simulink model "rpem_16_12_2005"  (Simulink 5.0)
settings: Solver=ode45  StartTime=0.0  StopTime=10.0  RelTol=1e-3
undefined symbols (not defined in the file): ts
libraries: simulink x7, dspmtrx3 x4, dspinverses x1, dsparch4 x1
settings Model: LastModifiedBy=LeO

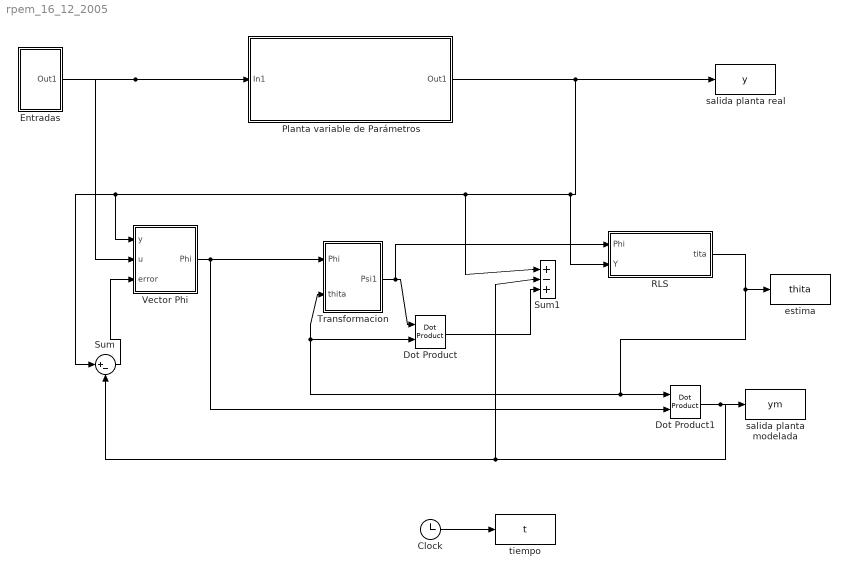
== system rpem_16_12_2005 ==
  Clock : Clock
      settings: Decimation=10
  Dot Product : simulink/Math Operations/Dot Product
  Dot Product1 : simulink/Math Operations/Dot Product
  Entradas : Subsystem
  Planta variable de Parámetros : Subsystem  mask{ruido=0.05, tiempo1=40}
      mask prompts: tiempo1 "tiempo de movimiento de parametros de la planta"
  RLS : Subsystem
  Sum : Sum  Inputs=|+-  SaturateOnIntegerOverflow=on
  Sum1 : Sum  Inputs=|+-+  SaturateOnIntegerOverflow=on
  Transformacion : Subsystem
  Vector Phi : Subsystem  mask{nu=1, ny=3, ne=1, nk=1}
      mask prompts: nu "Nº de u tomadas"; ny "Nº de y tomadas"; ne "Nº de errores tomados"; nk "Nº de retardo"
  estima : ToWorkspace  VariableName=thita  SampleTime=ts  SaveFormat=Array
  "salida planta modelada " : ToWorkspace  VariableName=ym  SampleTime=ts  SaveFormat=Array
  salida planta real : ToWorkspace  VariableName=y  SampleTime=ts  SaveFormat=Array
  "tiempo " : ToWorkspace  VariableName=t  SampleTime=ts  SaveFormat=Array
  wires:
  Entradas/1(Out1) -> Planta variable de Parámetros/1(In1), Vector Phi/2(u)
  Dot Product1/1 -> "salida planta modelada "/1, Sum/2, Sum1/2
  Clock/1 -> "tiempo "/1
  Planta variable de Parámetros/1(Out1) -> salida planta real/1, Vector Phi/1("y "), Sum/1, Sum1/1, RLS/2(Y)
  Transformacion/1(Psi1) -> Dot Product/1, RLS/1("Phi ")
  Vector Phi/1(Phi) -> Dot Product1/2, Transformacion/1(Phi)
  Sum/1 -> Vector Phi/3(error)
  RLS/1(tita) -> estima/1, Transformacion/2(thita), Dot Product/2, Dot Product1/1
  Dot Product/1 -> Sum1/3

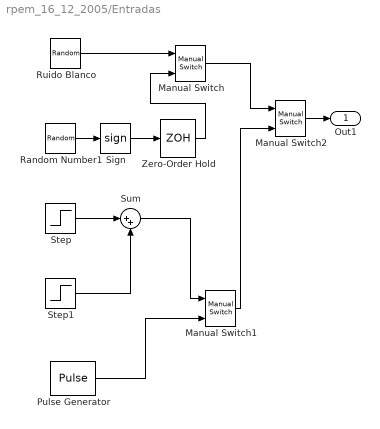
== system rpem_16_12_2005/Entradas ==
  Manual Switch : simulink/Signal Routing/Manual Switch  sw=1  action=0
  Manual Switch1 : simulink/Signal Routing/Manual Switch  sw=1  action=0
  Manual Switch2 : simulink/Signal Routing/Manual Switch  sw=1  action=0
  Pulse Generator : DiscretePulseGenerator  PulseType=Time based  PulseWidth=50
  Random Number1 : RandomNumber  SampleTime=0
  Ruido Blanco : RandomNumber  Variance=20  Seed=12  SampleTime=ts
  Sign : Signum
  Step : Step  Time=10  After=25  SampleTime=0.05
  Step1 : Step  Time=50  After=5  SampleTime=0.05
  Sum : Sum  Inputs=|++  SaturateOnIntegerOverflow=on
  Zero-Order Hold : ZeroOrderHold  SampleTime=0.05
  Out1 : Outport
  wires:
  Sign/1 -> Zero-Order Hold/1
  Random Number1/1 -> Sign/1
  Manual Switch/1 -> Manual Switch2/1
  Ruido Blanco/1 -> Manual Switch/1
  Zero-Order Hold/1 -> Manual Switch/2
  Manual Switch2/1 -> Out1/1
  Step/1 -> Sum/1
  Step1/1 -> Sum/2
  Manual Switch1/1 -> Manual Switch2/2
  Sum/1 -> Manual Switch1/1
  Pulse Generator/1 -> Manual Switch1/2

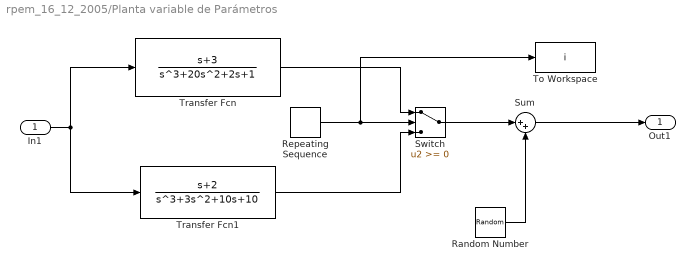
== system rpem_16_12_2005/Planta variable de Parámetros ==
  In1 : Inport
  Random Number : RandomNumber  Variance=ruido  SampleTime=0
  Repeating Sequence : simulink/Sources/Repeating Sequence  rep_seq_t=[0 2*tiempo1]  rep_seq_y=[1 -1 ]
  Sum : Sum  Inputs=|++  SaturateOnIntegerOverflow=on
  Switch : Switch  SaturateOnIntegerOverflow=on
  To Workspace : ToWorkspace  VariableName=i  SampleTime=-1  SaveFormat=Array
  Transfer Fcn : TransferFcn  Numerator=[1 3 ]  Denominator=[1 20 2 1]
  Transfer Fcn1 : TransferFcn  Numerator=[1 2]  Denominator=[1 3 10 10]
  Out1 : Outport
  wires:
  Transfer Fcn/1 -> Switch/1
  Repeating Sequence/1 -> Switch/2, To Workspace/1
  Transfer Fcn1/1 -> Switch/3
  In1/1 -> Transfer Fcn/1, Transfer Fcn1/1
  Switch/1 -> Sum/1
  Sum/1 -> Out1/1
  Random Number/1 -> Sum/2

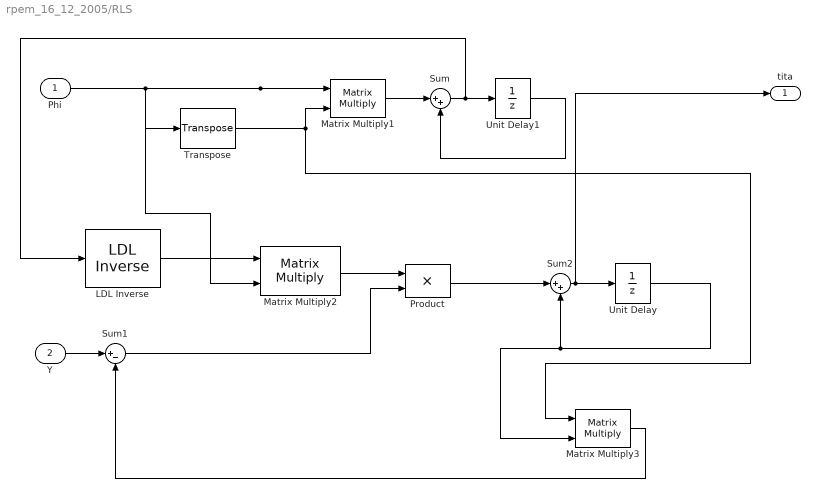
== system rpem_16_12_2005/RLS ==
  "Phi " : Inport  SampleTime=ts
  Y : Inport  Port=2  SampleTime=ts
  LDL Inverse : dspinverses/LDL Inverse  errmode=Ignore
  Matrix Multiply1 : dspmtrx3/Matrix Multiply  numInputPorts=2  OptimizationLevel=None
  Matrix Multiply2 : dspmtrx3/Matrix Multiply  numInputPorts=2  OptimizationLevel=None
  Matrix Multiply3 : dspmtrx3/Matrix Multiply  numInputPorts=2  OptimizationLevel=None
  Product : Product  SaturateOnIntegerOverflow=on
  Sum : Sum  Inputs=|++  SaturateOnIntegerOverflow=on
  Sum1 : Sum  Inputs=|+-  SaturateOnIntegerOverflow=on
  Sum2 : Sum  Inputs=|++  SaturateOnIntegerOverflow=on
  Transpose : dspmtrx3/Transpose  Hermitian=off
  Unit Delay : UnitDelay  X0=1*10^-3  SampleTime=ts
  Unit Delay1 : UnitDelay  X0=10^-3  SampleTime=ts
  tita : Outport
  wires:
  "Phi "/1 -> Transpose/1, Matrix Multiply2/2, Matrix Multiply1/1
  Transpose/1 -> Matrix Multiply3/1, Matrix Multiply1/2
  Matrix Multiply1/1 -> Sum/1
  Sum/1 -> Unit Delay1/1, LDL Inverse/1
  Unit Delay1/1 -> Sum/2
  LDL Inverse/1 -> Matrix Multiply2/1
  Sum2/1 -> Unit Delay/1, tita/1
  Y/1 -> Sum1/1
  Matrix Multiply2/1 -> Product/1
  Product/1 -> Sum2/1
  Matrix Multiply3/1 -> Sum1/2
  Sum1/1 -> Product/2
  Unit Delay/1 -> Matrix Multiply3/2, Sum2/2

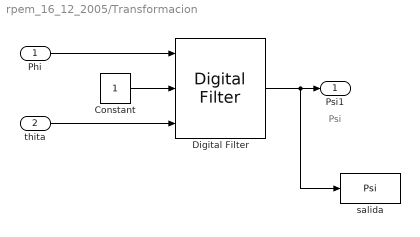
== system rpem_16_12_2005/Transformacion ==
  note: Psi
  Phi : Inport
  thita : Inport  Port=2
  Constant : Constant
  Digital Filter : dsparch4/Digital Filter  TypePopup=IIR (poles & zeros)  IIRFiltStruct=Direct form II transposed  AllPoleFiltStruct=Direct form  FIRFiltStruct=Direct form  CoeffSource=Input port(s)  NumCoeffs=[1 2]  DenCoeffs=[1 0.1]  BiQuadCoeffs=[1 0.3 0.4 1 0.1 0.2]  LatticeCoeffs=[0.2 0.4]  denIgnore=on  FiltPerSampPopup=One filter per frame  IC=0  ICnum=0  ICden=0
  salida : ToWorkspace  VariableName=Psi  SampleTime=ts  SaveFormat=Array
  Psi1 : Outport
  wires:
  Constant/1 -> Digital Filter/2
  Phi/1 -> Digital Filter/1
  thita/1 -> Digital Filter/3
  Digital Filter/1 -> Psi1/1, salida/1

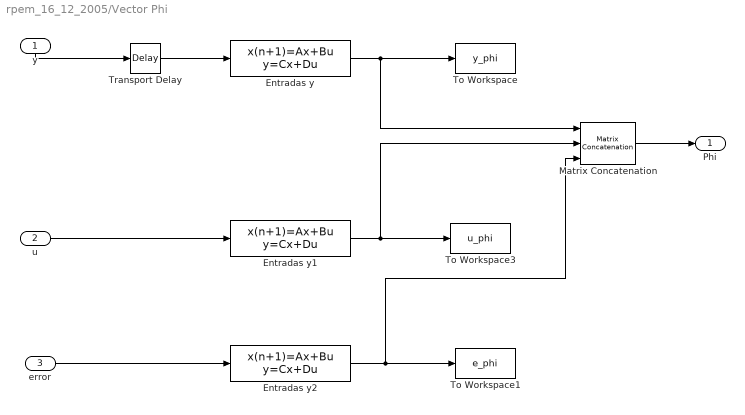
== system rpem_16_12_2005/Vector Phi ==
  "y " : Inport  Orientation=down  SampleTime=ts
  u : Inport  Port=2  SampleTime=ts
  error : Inport  Port=3  SampleTime=ts
  Entradas y : DiscreteStateSpace  A=[zeros(1,ny) ;eye(ny-1,ny)]  B=[[-1 zeros(1,ny-1)]']  C=[eye(ny)]  D=[zeros(1,ny)']  SampleTime=ts
  Entradas y1 : DiscreteStateSpace  A=[zeros(1,nu) ;eye(nu-1,nu)]  B=[[-1 zeros(1,nu-1)]']  C=[eye(nu)]  D=[zeros(1,nu)']  SampleTime=ts
  Entradas y2 : DiscreteStateSpace  A=[zeros(1,ne) ;eye(ne-1,ne)]  B=[[-1 zeros(1,ne-1)]']  C=[eye(ne)]  D=[zeros(1,ne)']  SampleTime=ts
  Matrix Concatenation : simulink/Math Operations/Matrix Concatenation  numInports=3  catMethod=Vertical
  To Workspace : ToWorkspace  VariableName=y_phi  SampleTime=ts  SaveFormat=Array
  To Workspace1 : ToWorkspace  VariableName=e_phi  SampleTime=ts  SaveFormat=Array
  To Workspace3 : ToWorkspace  VariableName=u_phi  SampleTime=ts  SaveFormat=Array
  Transport Delay : TransportDelay  DelayTime=nk*ts
  Phi : Outport
  wires:
  "y "/1 -> Transport Delay/1
  u/1 -> Entradas y1/1
  Entradas y/1 -> To Workspace/1, Matrix Concatenation/1
  Entradas y1/1 -> To Workspace3/1, Matrix Concatenation/2
  Matrix Concatenation/1 -> Phi/1
  Transport Delay/1 -> Entradas y/1
  error/1 -> Entradas y2/1
  Entradas y2/1 -> To Workspace1/1, Matrix Concatenation/3
